simulink library "myLibrary"  (R2023b)
settings: Solver=VariableStepAuto  StartTime=0.0  StopTime=10.0  RelTol=1e-3
undefined symbols (not defined in the file): Cac_n1, ctrl1, Da, Discrete, dtha, ee_sli_rtmsupport, FA, gcbh, Ha, Ini, init_DCline, init_IPC, init_line, init_load, init_SG, init_shunt, init_TH, init_trafo, init_VSC, initMachineBlocks, Ka, Lf, Llkd_pu, Llkq1_pu, magnitude, NET, P, plots_step, q0, Rac_n1, Radd, Rkd_pu, Rkq1_pu, Rload_add, sim_config, sps_rtmsupport, spsSteamTurbineModel, T_DC_NET, T_global, T_IPC, T_load, T_NET, T_SG, T_shunt, T_STATCOM, T_TH, T_trafo, T_VSC, Ts, tstep, Udiff_a, V1
libraries: spsSeriesRLCBranchLib x105, eeGeneralControl x72, $bdroot x70, spsCurrentMeasurementLib x48, spsParallelRLCBranchLib x39, spsVoltageMeasurementLib x33, spsControlledVoltageSourceLib x27, spsFirstOrderFilterLib x16, dspsigops x6, spsThreePhaseVIMeasurementLib x5, spsPLL3phLib x4, spsThreePhaseBreakerLib x3
(part 3 of 12)

== system myLibrary/SG_step ==
  Add : Sum  Inputs=-+
  Add1 : Sum
  Add2 : Sum  Inputs=+-
  Bus Selector : BusSelector  OutputSignals="Mechanical.Electromagnetic torque  Te (pu),dq0 components.Stator current  iq (pu),dq0 components.Stator current  id (pu),dq0 components.Field current  ifd (pu),dq0 components.Damper winding current  ikd (pu),dq0 components.Damper winding current  ikq1 (pu),dq0 components.Damper winding current  ikq2 (pu),dq0 components.Stator voltage  vq (pu),dq0 components.Stator voltage  vd (pu),Mechanical.Rotor angle deviation  d_theta (rad),Mechanical.Rotor speed  wm (pu),Mechanical.Rotor mechanical angle  theta (deg),Load angle   delta  (deg)"
  Constant4 : Constant  Value=[2/3 1/3; -1/3 1/3 ; -1/3 -2/3]
  Constant_pi1 : Constant  Value=pi/2
  Constant_pi2 : Constant  Value=-pi/2
  Current Measurement3 : spsCurrentMeasurementLib/Current Measurement  PhasorSimulation=off  OutputType=Complex  PSBequivalent=0
  Demux4 : Demux  Outputs=3
  Display : Display
  Display1 : Display
  Exciter : Subsystem
  Gain : Gain  Gain=T_SG.wb
  Gain1 : Gain  Gain=pi/180
  Gain2 : Gain  Gain=1/T_SG.Lmd_pu
  Gain3 : Gain  Gain=pi/180
  Governor-Turbine : Subsystem
  Integrator : Integrator
  Mux4 : Mux  Inputs=2
  PLL (3ph) : spsPLL3phLib/PLL (3ph)  Fmin=45  Par_Init=[0, 50]  ParK=[180, 3200, 1]  TcD=1e-4  MaxRateChangeFreq=12  FilterCutOffFreq=25  Ts=0  AGC=on
  PLL (3ph)1 : spsPLL3phLib/PLL (3ph)  Fmin=45  Par_Init=[initSG.theta_in, 50]  ParK=[180, 3200, 1]  TcD=1e-4  MaxRateChangeFreq=12  FilterCutOffFreq=25  Ts=0  AGC=on
  Pm : Step  Time=tstep_P  Before=initSG.Pm  After=initSG.Pm*(1+sim_config.DR)  SampleTime=1e-4
  SM1 : spsSynchronousMachinepuFundamentalLib/Synchronous Machine pu Fundamental  PresetModel=No  MechanicalLoad=Mechanical power Pm  ShowDetailedParameters=on  RotorType=Round  Units=per unit fundamental parameters  MeasurementBus=off  NominalParameters=initMachineBlocks{SGnum,1}  Stator=initMachineBlocks{SGnum,2}  Field=initMachineBlocks{SGnum,3}  Dampers2=initMachineBlocks{SGnum,4}  Dampers1="[ Rkd_pu   Llkd_pu  Rkq1_pu  Llkq1_pu]"  Mechanical=initMachineBlocks{SGnum,5}  PolePairs=1  InitialConditions=initMachineBlocks{SGnum,6}  SetSaturation=off  Saturation=[0.6404,0.7127,0.8441,0.9214,0.9956,1.082,1.19,1.316,1.457;0.7,0.7698,0.8872,0.9466,0.9969,1.046,1.1,1.151,1.201]  LoadFlowParameters=[1 5.55 0 0 0]  TsPowergui=0  TsBlock=-1  IterativeModel=Trapezoidal non iterative  IterativeDiscreteModel=Trapezoidal non iterative  BusType=PV  Pref=5.55  Qref=0  Qmin=-Inf  Qmax=Inf  PLF=0  QLF=0
  Scope{,1..2,4,6,10} (6 alike) : Scope
  Scope3 : Scope  NumInputPorts=3
  Scope5 : Scope  NumInputPorts=2
  Scope7 : Scope  NumInputPorts=2
  Series RLC Branch1 : spsSeriesRLCBranchLib/Series RLC Branch  LConnTagsString=__new0  RConnTagsString=__new0  BranchType=RL  Resistance=T_SG.Rtr*T_SG.Zbpu_l2g  Inductance=T_SG.Ltr*T_SG.Zbpu_l2g  SetiL0=off  InitialCurrent=initSG.Itr  Capacitance=P.C  Setx0=on  InitialVoltage=P.C  Measurements=None
  Series RLC Branch2 : PMComponent  DialogController=POWERSYS.PowerSysDialog  LoadFcn=sps_rtmsupport('LoadFcn',gcbh);  StartFcn=sps_rtmsupport('StartFcn',gcbh);  StopFcn=sps_rtmsupport('StopFcn',gcbh);  PhysicalDomain=powersysdomain  LeftPortType=p1  RightPortType=p1  LConnTagsString=__new0  RConnTagsString=__new0  mask(Series RLC Branch){BranchType=RL, Resistance=T_SG.Rtr*T_SG.Zbpu_l2g, Inductance=T_SG.Ltr*T_SG.Zbpu_l2g, SetiL0=off, InitialCurrent=initSG.Itr, Capacitance=P.C, Setx0=on, InitialVoltage=P.C, Measurements=None}
      mask prompts: BranchType "Branch type:"; Resistance "Resistance (Ohms):"; Inductance "Inductance (H):"; SetiL0 "Set the initial inductor current"; InitialCurrent "Inductor initial current (A):"; Capacitance "Capacitance (F):"; Setx0 "Set the initial capacitor voltage"; InitialVoltage "Capacitor initial voltage (V):"
      mask help:
      | Implements a series branch of RLC elements.
      | Use the 'Branch type' parameter to add or remove elements from the branch.
      mask init:
      | [s1,s2,s3,s4,r1,r2,l1,l2,c1,c2,c3,c4] = powericon('Series RLC Branch',Resistance,Inductance,Capacitance,BranchType);
      | powericon('RLCCback',gcb)
      | power_initmask();
      settings: LibrarySourceBlock=spsSeriesRLCBranchLib/Series RLC Branch  CopyFcn=sps_rtmsupport('CopyFcn',gcbh);  DeleteFcn=sps_rtmsupport('DeleteFcn',gcbh);  UndoDeleteFcn=sps_rtmsupport('UndoDeleteFcn',gcbh);  ModelCloseFcn=sps_rtmsupport('ModelCloseFcn',gcbh);  PreSaveFcn=sps_rtmsupport('PreSaveFcn',gcbh);  PostSaveFcn=sps_rtmsupport('PostSaveFcn',gcbh);  NameChangeFcn=sps_rtmsupport('NameChangeFcn',gcbh);  PreCopyFcn=sps_rtmsupport('PreCopyFcn',gcbh);  OpenFcn=sps_rtmsupport('OpenFcn',gcbh, [1 4 7 9]);  CloseFcn=sps_rtmsupport('CloseFcn',gcbh);  PreDeleteFcn=sps_rtmsupport('PreDeleteFcn',gcbh);
      mask Help: helpview(psbhelp);
      mask TypeOptions BranchType: RLC | R | L | C | RL | RC | LC | Open circuit
      mask Callback BranchType: powericon('RLCCback',gcb)
      mask Callback Resistance: powericon('RLCCback',gcb)
      mask Callback Inductance: powericon('RLCCback',gcb)
      mask Callback SetiL0: powericon('RLCCback',gcb)
      mask Callback Capacitance: powericon('RLCCback',gcb)
      mask Callback Setx0: powericon('RLCCback',gcb)
      mask TypeOptions Measurements: None | Branch voltage | Branch current | Branch voltage and current
      mask Display:
      | plot(s1,s2,s3,s4,r1,r2*1.5,l1,l2*1.5,c1,c2*1.5,c3,c4*1.5)
      | color('red')
      | port_label('LConn',1,'+')
  Series RLC Branch3 : PMComponent  DialogController=POWERSYS.PowerSysDialog  LoadFcn=sps_rtmsupport('LoadFcn',gcbh);  StartFcn=sps_rtmsupport('StartFcn',gcbh);  StopFcn=sps_rtmsupport('StopFcn',gcbh);  PhysicalDomain=powersysdomain  LeftPortType=p1  RightPortType=p1  LConnTagsString=__new0  RConnTagsString=__new0  mask(Series RLC Branch){BranchType=RL, Resistance=T_SG.Rtr*T_SG.Zbpu_l2g, Inductance=T_SG.Ltr*T_SG.Zbpu_l2g, SetiL0=off, InitialCurrent=initSG.Itr, Capacitance=P.C, Setx0=on, InitialVoltage=P.C, Measurements=None}
      mask prompts: BranchType "Branch type:"; Resistance "Resistance (Ohms):"; Inductance "Inductance (H):"; SetiL0 "Set the initial inductor current"; InitialCurrent "Inductor initial current (A):"; Capacitance "Capacitance (F):"; Setx0 "Set the initial capacitor voltage"; InitialVoltage "Capacitor initial voltage (V):"
      mask help:
      | Implements a series branch of RLC elements.
      | Use the 'Branch type' parameter to add or remove elements from the branch.
      mask init:
      | [s1,s2,s3,s4,r1,r2,l1,l2,c1,c2,c3,c4] = powericon('Series RLC Branch',Resistance,Inductance,Capacitance,BranchType);
      | powericon('RLCCback',gcb)
      | power_initmask();
      settings: LibrarySourceBlock=spsSeriesRLCBranchLib/Series RLC Branch  CopyFcn=sps_rtmsupport('CopyFcn',gcbh);  DeleteFcn=sps_rtmsupport('DeleteFcn',gcbh);  UndoDeleteFcn=sps_rtmsupport('UndoDeleteFcn',gcbh);  ModelCloseFcn=sps_rtmsupport('ModelCloseFcn',gcbh);  PreSaveFcn=sps_rtmsupport('PreSaveFcn',gcbh);  PostSaveFcn=sps_rtmsupport('PostSaveFcn',gcbh);  NameChangeFcn=sps_rtmsupport('NameChangeFcn',gcbh);  PreCopyFcn=sps_rtmsupport('PreCopyFcn',gcbh);  OpenFcn=sps_rtmsupport('OpenFcn',gcbh, [1 4 7 9]);  CloseFcn=sps_rtmsupport('CloseFcn',gcbh);  PreDeleteFcn=sps_rtmsupport('PreDeleteFcn',gcbh);
      mask Help: helpview(psbhelp);
      mask TypeOptions BranchType: RLC | R | L | C | RL | RC | LC | Open circuit
      mask Callback BranchType: powericon('RLCCback',gcb)
      mask Callback Resistance: powericon('RLCCback',gcb)
      mask Callback Inductance: powericon('RLCCback',gcb)
      mask Callback SetiL0: powericon('RLCCback',gcb)
      mask Callback Capacitance: powericon('RLCCback',gcb)
      mask Callback Setx0: powericon('RLCCback',gcb)
      mask TypeOptions Measurements: None | Branch voltage | Branch current | Branch voltage and current
      mask Display:
      | plot(s1,s2,s3,s4,r1,r2*1.5,l1,l2*1.5,c1,c2*1.5,c3,c4*1.5)
      | color('red')
      | port_label('LConn',1,'+')
  Sum : Sum  Inputs=++++
  Te : Scope
  Three-Phase Series RLC Branch4 : spsThreePhaseSeriesRLCBranchLib/Three-Phase Series RLC Branch  LConnTagsString=A|B|C  RConnTagsString=A|B|C  BranchType=R  Resistance=T_SG.Rsnb*T_SG.Zbpu_l2g  Inductance=NET.L1_2/2  Capacitance=1/0.0528/(2*pi*50)  Measurements=None
  Three-Phase V-I Measurement : spsThreePhaseVIMeasurementLib/Three-Phase V-I Measurement  VoltageMeasurement=phase-to-phase  SetLabelV=off  LabelV=Vpcc  Vpu=off  VpuLL=off  CurrentMeasurement=no  SetLabelI=off  LabelI=Iabc  Ipu=off  Pbase=100e6  Vbase=500e3  OutputType=Complex  PhasorSimulation=off  PSBequivalent=0
  Three-Phase V-I Measurement1 : spsThreePhaseVIMeasurementLib/Three-Phase V-I Measurement  VoltageMeasurement=phase-to-phase  SetLabelV=off  LabelV=Vtr  Vpu=off  VpuLL=off  CurrentMeasurement=no  SetLabelI=off  LabelI=Iabc  Ipu=off  Pbase=100e6  Vbase=500e3  OutputType=Complex  PhasorSimulation=off  PSBequivalent=0
  Unwrap : dspsigops/Unwrap  tol=pi  InputProcessing=Columns as channels (frame based)  running=off
  Unwrap1 : dspsigops/Unwrap  tol=pi  InputProcessing=Columns as channels (frame based)  running=off
  Unwrap2 : dspsigops/Unwrap  tol=pi  InputProcessing=Columns as channels (frame based)  running=off
  "Vector magnitude " : Subsystem
  Vf : Constant  Value=initSG.Vf
  deg2rad : Gain  Gain=pi/180
  isqd : Scope  NumInputPorts=2
  mtx4 : Product  Multiplication=Matrix(*)
  qd3 : $bdroot/qd transform  SystemSampleTime=-1  VariantActivationTime=update diagram  AllowFlexibleInterface=on  Latency=0  AutoFrameSizeCalculation=off
  v_ref : Step  Time=tstep_V  Before=initSG.Vref  After=initSG.Vref*(1+sim_config.DR)  SampleTime=1e-4
  vqd : Scope  NumInputPorts=3
  A : PMIOPort  Side=Right
  B : PMIOPort  Port=2  Side=Right
  C : PMIOPort  Port=3  Side=Right
  tag scope: V_fn_pcc=global, theta_SG1=global, w_SG1=global
  wires:
  Three-Phase V-I Measurement1/1 -> [Vtr]
  Three-Phase V-I Measurement/1 -> [Vpcc]
  Bus Selector/10 -> [d_theta], Add1/1, Scope/1  "<Rotor angle deviation  d_theta (rad)>"
  Bus Selector/7 -> [ikq2]  "<Damper winding current  ikq2 (pu)>"
  [Vtr] -> PLL (3ph)/1
  Gain2/1 -> Scope1/1, [ifd]
  Bus Selector/5 -> [ikd]  "<Damper winding current  ikd (pu)>"
  Bus Selector/3 -> isqd/2, [isd]  "<Stator current  id (pu)>"
  Bus Selector/11 -> [we], Gain/1  "<Rotor speed  wm (pu)>"
  Bus Selector/6 -> [ikq1]  "<Damper winding current  ikq1 (pu)>"
  [Vpcc] -> PLL (3ph)1/1
  Bus Selector/4 -> Gain2/1  "<Field current  ifd (pu)>"
  Bus Selector/8 -> "Vector magnitude "/1(Vq), vqd/1, [vq]  "<Stator voltage  vq (pu)>"
  Bus Selector/1 -> Te/1, [Te]  "<Electromagnetic torque  Te (pu)>"
  Bus Selector/9 -> "Vector magnitude "/2(Vd), vqd/2, [vd]  "<Stator voltage  vd (pu)>"
  Gain/1 -> Scope6/1, [w_SG1], Integrator/1
  Current Measurement3/1 -> Scope2/1  "a"
  "Vector magnitude "/1(V) -> vqd/3  "V"
  Unwrap1/1 -> Add/1
  SM1/1 -> Bus Selector/1
  Bus Selector/13 -> [delta], Gain1/1, Gain3/1  "<Load angle   delta  (deg)>"
  Bus Selector/12 -> deg2rad/1, [theta]  "<Rotor mechanical angle  theta (deg)>"
  Bus Selector/2 -> isqd/1, [isq]  "<Stator current  iq (pu)>"
  Add/1 -> Scope4/1, Sum/4  "theta_in"
  Integrator/1 -> Sum/2
  PLL (3ph)1/2 -> Unwrap/1
  PLL (3ph)/2 -> Unwrap1/1
  Unwrap/1 -> Add/2
  Constant_pi1/1 -> Add1/2
  Add1/1 -> Scope5/1  "d_theta"
  Gain3/1 -> Scope5/2  "load_angle"
  Gain1/1 -> Sum/3
  Constant_pi2/1 -> Sum/1
  Governor-Turbine/1(Pm) -> SM1/1
  [we] -> Governor-Turbine/2(wm)  "wm"
  Pm/1 -> Governor-Turbine/1(Pref)
  [d_theta] -> Governor-Turbine/3(d_theta)
  deg2rad/1 -> Unwrap2/1
  Unwrap2/1 -> Add2/2, Scope3/3, [theta_SG1]  "THETA MATLAB"
  [we] -> Exciter/4(Vsi1)
  [vd] -> Exciter/3(Vd)
  [ifd] -> Exciter/6(Ifd_pu)
  [Te] -> Exciter/5(Vsi2)
  Vf/1 -> Exciter/7(Efd0_pu)
  v_ref/1 -> Exciter/1(V_REF)
  Exciter/1(Out1) -> SM1/2
  [vq] -> Exciter/2(Vq)
  Sum/1 -> Scope3/2, Add2/1  "OUR CALC"
  Add2/1 -> Scope3/1  "RESTA"
  qd3/1 -> Display/1, Scope7/1
  Demux4/1 -> Mux4/1
  [Vpcc] -> Demux4/1
  [V_fn_pcc] -> qd3/1
  Constant4/1 -> mtx4/1
  Demux4/2 -> Mux4/2
  Mux4/1 -> mtx4/2
  mtx4/1 -> [V_fn_pcc], Scope10/1
  qd3/2 -> Display1/1, Scope7/2
  [theta_SG1] -> qd3/2
  connections:
  Three-Phase V-I Measurement/LConn3 -- SM1/RConn3
  SM1/RConn2 -- Three-Phase V-I Measurement/LConn2
  Three-Phase V-I Measurement/LConn1 -- SM1/RConn1
  B/RConn1 -- Three-Phase V-I Measurement1/RConn2
  Series RLC Branch3/RConn1 -- Three-Phase V-I Measurement1/LConn3
  Series RLC Branch1/RConn1 -- Three-Phase V-I Measurement1/LConn1
  Current Measurement3/RConn1 -- Three-Phase Series RLC Branch4/RConn1
  A/RConn1 -- Three-Phase V-I Measurement1/RConn1
  C/RConn1 -- Three-Phase V-I Measurement1/RConn3
  Series RLC Branch2/RConn1 -- Three-Phase V-I Measurement1/LConn2
  Three-Phase V-I Measurement/RConn1 -- Series RLC Branch1/LConn1 -- Current Measurement3/LConn1
  Three-Phase V-I Measurement/RConn3 -- Series RLC Branch3/LConn1 -- Three-Phase Series RLC Branch4/RConn3
  Three-Phase Series RLC Branch4/LConn3 -- Three-Phase Series RLC Branch4/LConn2 -- Three-Phase Series RLC Branch4/LConn1
  Three-Phase V-I Measurement/RConn2 -- Series RLC Branch2/LConn1 -- Three-Phase Series RLC Branch4/RConn2

== system myLibrary/STATCOM ==
  Constant5 : Constant  Value=[ 2/3 1/3; -1/3 1/3 ; -1/3 -2/3]
  Control : Subsystem
      settings: PortSchema="{\"entries\":[{\"content\":{\"sides\":[{\"content\":{},\"type\":\"ConnectorPlacement.EquallySpacedRectSide\",\"uuid\":\"681c0b5f-022d-4b6d-8fe2-73940743a76e\"},{\"content\":{\"side\":\"RIGHT\"},\"type\":\"ConnectorPlacement.EquallySpacedRectSide\",\"uuid\":\"e9b400c8-e13f-4caf-91a1-f348979675fd\"},{\"content\":{\"connectorIds\":[\"In1\",\"Out1\",\"Out2\"],\"side\":\"TOP\"},\"type\":\"ConnectorPlacement.EquallySpacedRectSide\",\"uuid\":\"348007cb-ce67-4c45-ad7b-36ba89db6185\"},{\"content\":{\"connectorIds\":[\"In2\",\"In3\",\"In4\"],\"side\":\"BOTTOM\"},\"type\":\"ConnectorPlacement.EquallySpacedRectSide\",\"uuid\":\"fd6a847a-5d69-44cd-a0d1-495126761350\"}]},\"type\":\"ConnectorPlacement.EquallySpacedConnector\",\"uuid\":\"d16b8cae-5ced-4c76-a87e-983e154fb48f\"}],\"packageUris\":[\"http://schema.mathworks.com/mf0/Connector/R2020b\"],\"version\":\"1.0\"}"
  Current Measurement20 : spsCurrentMeasurementLib/Current Measurement  PhasorSimulation=off  OutputType=Complex  PSBequivalent=0
  Current Measurement21 : spsCurrentMeasurementLib/Current Measurement  PhasorSimulation=off  OutputType=Complex  PSBequivalent=0
  Current Measurement25 : spsCurrentMeasurementLib/Current Measurement  PhasorSimulation=off  OutputType=Complex  PSBequivalent=0
  Electrical : Subsystem
  Ig_l2g : Gain  Gain=1/T_VSC.Ibpu_l2g
  Is_l2g : Gain  Gain=1/T_VSC.Ibpu_l2g
  Mux10 : Mux  Inputs=2
  Mux4 : Mux  Inputs=3
  Product4 : Product  Multiplication=Matrix(*)
  Scope : Scope  NumInputPorts=3
  Series RLC Branch1 : spsSeriesRLCBranchLib/Series RLC Branch  LConnTagsString=__new0  RConnTagsString=__new0  BranchType=RL  Resistance=initVSC.Rtr  Inductance=initVSC.Ltr  SetiL0=off  InitialCurrent=initVSC.Iga  Capacitance=P.C  Setx0=on  InitialVoltage=P.C  Measurements=None
  Series RLC Branch10 : spsSeriesRLCBranchLib/Series RLC Branch  LConnTagsString=__new0  RConnTagsString=__new0  BranchType=R  Resistance=initVSC.Rac  Inductance=Lf  SetiL0=off  InitialCurrent=0  Capacitance=Cac_n1  Setx0=on  InitialVoltage=vcini_n1  Measurements=None
  Series RLC Branch2 : spsSeriesRLCBranchLib/Series RLC Branch  LConnTagsString=__new0  RConnTagsString=__new0  BranchType=RL  Resistance=initVSC.Rtr  Inductance=initVSC.Ltr  SetiL0=on  InitialCurrent=initVSC.Igb  Capacitance=P.C  Setx0=on  InitialVoltage=P.C  Measurements=None
  Series RLC Branch3 : spsSeriesRLCBranchLib/Series RLC Branch  LConnTagsString=__new0  RConnTagsString=__new0  BranchType=RL  Resistance=initVSC.Rtr  Inductance=initVSC.Ltr  SetiL0=on  InitialCurrent=initVSC.Igc  Capacitance=P.C  Setx0=on  InitialVoltage=P.C  Measurements=None
  Series RLC Branch4 : spsSeriesRLCBranchLib/Series RLC Branch  LConnTagsString=__new0  RConnTagsString=__new0  BranchType=C  Resistance=Rac_n1  Inductance=Lf  SetiL0=off  InitialCurrent=0  Capacitance=initVSC.Cac  Setx0=on  InitialVoltage=initVSC.Ucap_b  Measurements=None
  Series RLC Branch5 : spsSeriesRLCBranchLib/Series RLC Branch  LConnTagsString=__new0  RConnTagsString=__new0  BranchType=C  Resistance=Rac_n1  Inductance=Lf  SetiL0=off  InitialCurrent=0  Capacitance=initVSC.Cac  Setx0=on  InitialVoltage=initVSC.Ucap_a  Measurements=None
  Series RLC Branch6 : spsSeriesRLCBranchLib/Series RLC Branch  LConnTagsString=__new0  RConnTagsString=__new0  BranchType=R  Resistance=initVSC.Rac  Inductance=Lf  SetiL0=off  InitialCurrent=0  Capacitance=Cac_n1  Setx0=on  InitialVoltage=vcini_n1  Measurements=None
  Series RLC Branch8 : spsSeriesRLCBranchLib/Series RLC Branch  LConnTagsString=__new0  RConnTagsString=__new0  BranchType=R  Resistance=initVSC.Rac  Inductance=Lf  SetiL0=off  InitialCurrent=0  Capacitance=Cac_n1  Setx0=on  InitialVoltage=vcini_n1  Measurements=None
  Series RLC Branch9 : spsSeriesRLCBranchLib/Series RLC Branch  LConnTagsString=__new0  RConnTagsString=__new0  BranchType=C  Resistance=Rac_n1  Inductance=Lf  SetiL0=off  InitialCurrent=0  Capacitance=initVSC.Cac  Setx0=on  InitialVoltage=initVSC.Ucap_c  Measurements=None
  U_g2l : Gain  Gain=1/T_VSC.Vbpu_l2g
  Vdiff_l2g : Gain  Gain=T_VSC.Vbpu_l2g
  Voltage Measurement{,1..4} (5 alike) : spsVoltageMeasurementLib/Voltage Measurement  PhasorSimulation=off  OutputType=Complex  PSBequivalent=0
  VA : PMIOPort  Side=Right
  VB : PMIOPort  Port=2  Side=Right
  VC : PMIOPort  Port=3  Side=Right
  wires:
  Voltage Measurement1/1 -> Mux10/2
  Constant5/1 -> Product4/1
  Mux10/1 -> Product4/2
  Voltage Measurement/1 -> Mux10/1
  Product4/1 -> U_g2l/1
  Control/1(Vdiff_abc) -> Vdiff_l2g/1
  Electrical/2(Is) -> Is_l2g/1
  Vdiff_l2g/1 -> Electrical/2(vdiff)
  Is_l2g/1 -> Control/3(Iss)
  U_g2l/1 -> Control/2(U)
  Current Measurement20/1 -> Mux4/2
  Current Measurement21/1 -> Mux4/1
  Mux4/1 -> Ig_l2g/1
  Current Measurement25/1 -> Mux4/3
  Ig_l2g/1 -> Control/1(ig_abc)
  Voltage Measurement3/1 -> Scope/2
  Voltage Measurement2/1 -> Scope/1
  Voltage Measurement4/1 -> Scope/3
  Control/2(Pac) -> Electrical/1(Pac)
  Electrical/1(Vdc) -> Control/4(Vdc)
  connections:
  VB/RConn1 -- Current Measurement20/RConn1
  Series RLC Branch1/LConn1 -- Series RLC Branch5/LConn1 -- Voltage Measurement2/LConn1 -- Voltage Measurement/LConn1 -- Electrical/LConn1
  Voltage Measurement1/LConn2 -- Series RLC Branch9/LConn1 -- Voltage Measurement4/LConn1 -- Series RLC Branch3/LConn1 -- Electrical/LConn3
  VA/RConn1 -- Current Measurement21/RConn1
  Voltage Measurement1/LConn1 -- Series RLC Branch4/LConn1 -- Voltage Measurement3/LConn1 -- Series RLC Branch2/LConn1 -- Voltage Measurement/LConn2 -- Electrical/LConn2
  Current Measurement25/RConn1 -- VC/RConn1
  Series RLC Branch1/RConn1 -- Current Measurement21/LConn1
  Series RLC Branch2/RConn1 -- Current Measurement20/LConn1
  Series RLC Branch3/RConn1 -- Current Measurement25/LConn1
  Voltage Measurement2/LConn2 -- Series RLC Branch6/LConn1 -- Series RLC Branch5/RConn1
  Voltage Measurement3/LConn2 -- Series RLC Branch4/RConn1 -- Series RLC Branch8/LConn1
  Voltage Measurement4/LConn2 -- Series RLC Branch10/LConn1 -- Series RLC Branch9/RConn1
  Series RLC Branch10/RConn1 -- Series RLC Branch8/RConn1 -- Series RLC Branch6/RConn1

== system myLibrary/TH ==
  note: Grid Thevenin
  Series RLC Branch : spsSeriesRLCBranchLib/Series RLC Branch  LConnTagsString=__new0  RConnTagsString=__new0  BranchType=RL  Resistance=T.R  Inductance=T.L  SetiL0=off  InitialCurrent=ini.Itha  Capacitance=1e-6  Setx0=off  InitialVoltage=0  Measurements=None
  Series RLC Branch1 : spsSeriesRLCBranchLib/Series RLC Branch  LConnTagsString=__new0  RConnTagsString=__new0  BranchType=RL  Resistance=T.R  Inductance=T.L  SetiL0=on  InitialCurrent=ini.Ithb  Capacitance=1e-6  Setx0=off  InitialVoltage=0  Measurements=None
  Series RLC Branch2 : spsSeriesRLCBranchLib/Series RLC Branch  LConnTagsString=__new0  RConnTagsString=__new0  BranchType=RL  Resistance=T.R  Inductance=T.L  SetiL0=on  InitialCurrent=ini.Ithc  Capacitance=1e-6  Setx0=off  InitialVoltage=0  Measurements=None
  Three-Phase Source : spsThreePhaseSourceLib/Three-Phase Source  InternalConnection=Y  VoltagePhases=off  Voltage=ini.Vmag  PhaseAngle=ini.angle*180/pi  Voltage_phases=[25e3 25e3 25e3]/sqrt(3)  PhaseAngles_phases=[0 -120 +120]  Frequency="T_global{T_global.Area == T.Area,\"fb\"}"  NonIdealSource=off  SpecifyImpedance=off  Resistance=0.8929  Inductance=16.58e-3  ShortCircuitLevel=100e6  BaseVoltage=25e3  XRratio=7  BusType=swing  Pref=10e3  Qref=0  Prefabc=[10e3, 10e3, 10e3]  Qrefabc=[0, 0, 0]  Qmin=-inf  Qmax=inf
  A : PMIOPort  Side=Right
  B : PMIOPort  Port=2  Side=Right
  C : PMIOPort  Port=3  Side=Right
  connections:
  Series RLC Branch1/LConn1 -- Three-Phase Source/RConn2
  Series RLC Branch/LConn1 -- Three-Phase Source/RConn1
  A/RConn1 -- Series RLC Branch/RConn1
  B/RConn1 -- Series RLC Branch1/RConn1
  Series RLC Branch2/LConn1 -- Three-Phase Source/RConn3
  C/RConn1 -- Series RLC Branch2/RConn1

== system myLibrary/TH_step ==
  note: Grid Thevenin
  Constant1 : Constant  Value="2*pi*T_global{T_global.Area == T.Area,\"fb\"}"
  Constant2 : Constant  Value=2*pi/3
  Controlled Voltage Source : spsControlledVoltageSourceLib/Controlled Voltage Source  Initialize=on  Source_Type=AC  Amplitude=ini.Vmag/sqrt(3)*sqrt(2)  Phase=ini.angle*180/pi  Frequency=T_global.f_Hz  Measurements=None
  Controlled Voltage Source3 : spsControlledVoltageSourceLib/Controlled Voltage Source  Initialize=on  Source_Type=AC  Amplitude=ini.Vmag/sqrt(3)*sqrt(2)  Phase=ini.angle*180/pi-120  Frequency=T_global.f_Hz  Measurements=None
  Controlled Voltage Source4 : spsControlledVoltageSourceLib/Controlled Voltage Source  Initialize=on  Source_Type=AC  Amplitude=ini.Vmag/sqrt(3)*sqrt(2)  Phase=ini.angle*180/pi+120  Frequency=T_global.f_Hz  Measurements=None
  Current Measurement : spsCurrentMeasurementLib/Current Measurement  PhasorSimulation=off  OutputType=Complex  PSBequivalent=0
  Current Measurement1 : spsCurrentMeasurementLib/Current Measurement  PhasorSimulation=off  OutputType=Complex  PSBequivalent=0
  Current Measurement2 : spsCurrentMeasurementLib/Current Measurement  PhasorSimulation=off  OutputType=Complex  PSBequivalent=0
  Ground : spsGroundLib/Ground  LConnTagsString=a
  Integrator : Integrator  InitialCondition=ini.angle
  Product : Product
  Product1 : Product
  Product2 : Product
  Scope1 : Scope
  Scope2 : Scope
  Scope3 : Scope  NumInputPorts=3
  Series RLC Branch : spsSeriesRLCBranchLib/Series RLC Branch  LConnTagsString=__new0  RConnTagsString=__new0  BranchType=RL  Resistance=T.R  Inductance=T.L  SetiL0=on  InitialCurrent=ini.Itha  Capacitance=1e-6  Setx0=off  InitialVoltage=0  Measurements=None
  Series RLC Branch1 : spsSeriesRLCBranchLib/Series RLC Branch  LConnTagsString=__new0  RConnTagsString=__new0  BranchType=RL  Resistance=T.R  Inductance=T.L  SetiL0=on  InitialCurrent=ini.Ithb  Capacitance=1e-6  Setx0=off  InitialVoltage=0  Measurements=None
  Series RLC Branch2 : spsSeriesRLCBranchLib/Series RLC Branch  LConnTagsString=__new0  RConnTagsString=__new0  BranchType=RL  Resistance=T.R  Inductance=T.L  SetiL0=on  InitialCurrent=ini.Ithc  Capacitance=1e-6  Setx0=off  InitialVoltage=0  Measurements=None
  Sin : Trigonometry
  Sin1 : Trigonometry
  Sin2 : Trigonometry
  Step : Step  Time=tstep  Before=ini.Vmag/sqrt(3)*sqrt(2)  After=V1/sqrt(3)*sqrt(2)  SampleTime=1e-4
  Sum : Sum  Inputs=+-
  Sum1 : Sum
  Voltage Measurement : spsVoltageMeasurementLib/Voltage Measurement  PhasorSimulation=off  OutputType=Complex  PSBequivalent=0
  Voltage Measurement1 : spsVoltageMeasurementLib/Voltage Measurement  PhasorSimulation=off  OutputType=Complex  PSBequivalent=0
  A : PMIOPort  Side=Right
  B : PMIOPort  Port=2  Side=Right
  C : PMIOPort  Port=3  Side=Right
  wires:
  Current Measurement2/1 -> Scope3/3
  Current Measurement1/1 -> Scope3/2
  Current Measurement/1 -> Scope3/1
  Voltage Measurement1/1 -> Scope2/1
  Voltage Measurement/1 -> Scope1/1
  Sum1/1 -> Sin2/1
  Sin/1 -> Product/1
  Product1/1 -> Controlled Voltage Source3/1
  Product/1 -> Controlled Voltage Source/1
  Sum/1 -> Sin1/1
  Sin1/1 -> Product1/1
  Step/1 -> Product2/2, Product1/2, Product/2
  Sin2/1 -> Product2/1
  Product2/1 -> Controlled Voltage Source4/1
  Constant1/1 -> Integrator/1
  Constant2/1 -> Sum1/2, Sum/2
  Integrator/1 -> Sum/1, Sum1/1, Sin/1
  connections:
  Current Measurement2/RConn1 -- C/RConn1
  Voltage Measurement1/LConn2 -- Controlled Voltage Source3/RConn1 -- Series RLC Branch1/LConn1
  Voltage Measurement1/LConn1 -- Controlled Voltage Source/RConn1 -- Series RLC Branch/LConn1
  Current Measurement1/RConn1 -- B/RConn1 -- Voltage Measurement/LConn2
  Current Measurement/RConn1 -- A/RConn1 -- Voltage Measurement/LConn1
  Series RLC Branch/RConn1 -- Current Measurement/LConn1
  Series RLC Branch1/RConn1 -- Current Measurement1/LConn1
  Controlled Voltage Source4/RConn1 -- Series RLC Branch2/LConn1
  Series RLC Branch2/RConn1 -- Current Measurement2/LConn1
  Controlled Voltage Source/LConn1 -- Controlled Voltage Source4/LConn1 -- Ground/LConn1 -- Controlled Voltage Source3/LConn1

== system myLibrary/Trafo ==
  Series RLC Branch1 : spsSeriesRLCBranchLib/Series RLC Branch  LConnTagsString=__new0  RConnTagsString=__new0  BranchType=RL  Resistance=T.R  Inductance=T.L  SetiL0=on  InitialCurrent=ini.Ia  Capacitance=P.C  Setx0=on  InitialVoltage=P.C  Measurements=None
  Series RLC Branch2 : spsSeriesRLCBranchLib/Series RLC Branch  LConnTagsString=__new0  RConnTagsString=__new0  BranchType=RL  Resistance=T.R  Inductance=T.L  SetiL0=on  InitialCurrent=ini.Ib  Capacitance=P.C  Setx0=on  InitialVoltage=P.C  Measurements=None
  Series RLC Branch3 : spsSeriesRLCBranchLib/Series RLC Branch  LConnTagsString=__new0  RConnTagsString=__new0  BranchType=RL  Resistance=T.R  Inductance=T.L  SetiL0=on  InitialCurrent=ini.Ic  Capacitance=P.C  Setx0=on  InitialVoltage=P.C  Measurements=None
  A1 : PMIOPort  Side=Left
  B1 : PMIOPort  Port=2  Side=Left
  C1 : PMIOPort  Port=3  Side=Left
  A2 : PMIOPort  Port=4  Side=Right
  B2 : PMIOPort  Port=5  Side=Right
  C2 : PMIOPort  Port=6  Side=Right
  connections:
  Series RLC Branch1/RConn1 -- A2/RConn1
  Series RLC Branch2/RConn1 -- B2/RConn1
  Series RLC Branch3/RConn1 -- C2/RConn1
  Series RLC Branch2/LConn1 -- B1/RConn1
  Series RLC Branch1/LConn1 -- A1/RConn1
  Series RLC Branch3/LConn1 -- C1/RConn1

== system myLibrary/qd transform ==
  abc : Inport
  angle : Inport  Port=2
  Demux8 : Demux  Outputs=3
  qd0 Transformation : Subsystem
  q : Outport
  d : Outport  Port=2
  wires:
  qd0 Transformation/1(q) -> q/1  "q"
  Demux8/1 -> qd0 Transformation/1(a)
  qd0 Transformation/2(d) -> d/1  "d"
  Demux8/2 -> qd0 Transformation/2(b)
  abc/1 -> Demux8/1
  Demux8/3 -> qd0 Transformation/3(c)
  angle/1 -> qd0 Transformation/4(Angle)

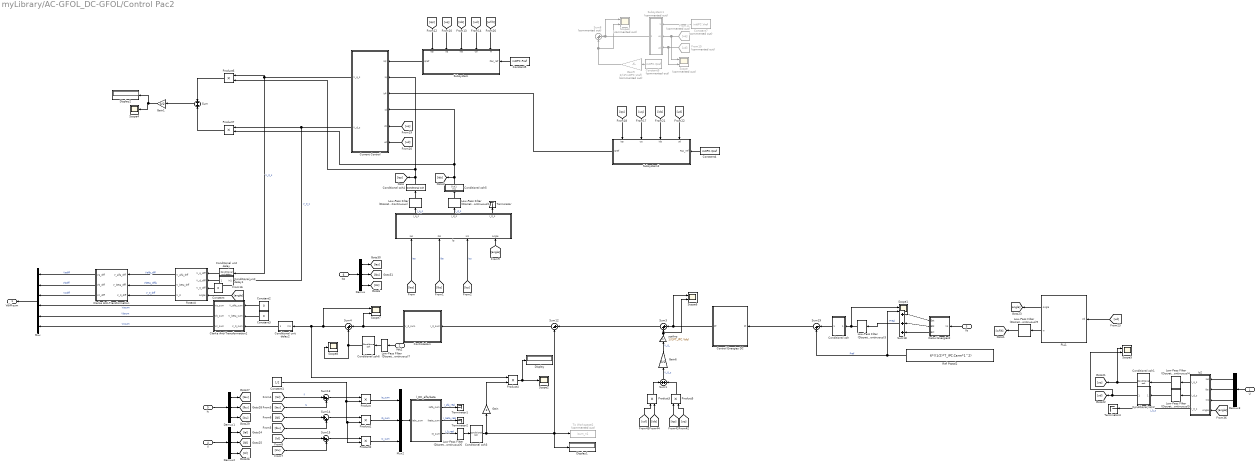
== system myLibrary/AC-GFOL_DC-GFOL/Control Pac2 ==
  U : Inport
  Vdc2 : Inport  Port=2
  Vs : Inport  Port=3
  Il : Inport  Port=4
  Iu : Inport  Port=5
  Iss : Inport  Port=6
  Calcul Energies2 : Subsystem
  Clarke Anti-Transformation : Subsystem
  Clarke Anti-Transformation2 : Subsystem
  Conditional unit delay : $bdroot/GFOL/Control/Conditional unit delay  SystemSampleTime=-1  VariantActivationTime=update diagram  AllowFlexibleInterface=on  Latency=0  AutoFrameSizeCalculation=off
      link override Constant4: Value=T_IPC.tau_cmd
      link override Unit Delay2: InitialCondition=initIPC.vdiffq  SampleTime=T_IPC.tau_cmd
  Conditional unit delay1 : Subsystem
  Conditional unit delay2 : Subsystem
  Conditional zoh : Subsystem
  Conditional zoh{1,3..4,6} (4 alike) : $bdroot/AC-GFOL_DC-GFOL/Control Pac2/Conditional zoh  SystemSampleTime=-1  VariantActivationTime=update diagram  AllowFlexibleInterface=on  Latency=0  AutoFrameSizeCalculation=off
  Conditional zoh2 : Subsystem
  Conditional zoh5 : Subsystem
  Constant : Constant  Value=0
  Constant1 : Constant  Value=1/2
  Constant2 : Constant  Value=0
  Constant3 : Constant  Value=0
  Constant4 : Constant  Value=initIPC.Qref
  Constant5 : Constant  Value=initIPC.Pref
  Constant7 : Constant  Commented=on  Value=initIPC.Vref
  Constant9 : Constant  Commented=on  Value=initIPC.Qref
  Control Energies DC : Subsystem
  Controladors : Subsystem
  Current Control : Subsystem
  Demux{,1..3} (4 alike) : Demux  Outputs=3
  Display : Display
  Display1 : Display
  Display2 : Display
  From11 : From  Commented=on  GotoTag=uq
  From15 : From  Commented=on  GotoTag=ud
  Gain : Gain  Gain=3
  Gain1 : Gain  Gain=3/2
  Gain6 : Gain  Gain=3/2
  Gain9 : Gain  Commented=on  Gain=2/(3*initIPC.Vref)
  Is : Subsystem
  Is2 : Subsystem
  Low-Pass Filter (Discrete or Continuous) : eeGeneralControl/Low-Pass Filter (Discrete or Continuous)  K=1  T=T_IPC.delay  B=inf  A=-inf  init_option=Specify as parameter  x0=initIPC.idiffq  Ts=0
  Low-Pass Filter (Discrete or Continuous)1 : eeGeneralControl/Low-Pass Filter (Discrete or Continuous)  K=1  T=T_IPC.delay  B=inf  A=-inf  init_option=Specify as parameter  x0=initIPC.idiffd  Ts=0
  Low-Pass Filter (Discrete or Continuous)3 : eeGeneralControl/Low-Pass Filter (Discrete or Continuous)  K=1  T=T_IPC.delay  B=inf  A=-inf  init_option=Specify as parameter  x0=6*((1/2)*T_IPC.Carm*1^2)  Ts=0
  Low-Pass Filter (Discrete or Continuous)4 : eeGeneralControl/Low-Pass Filter (Discrete or Continuous)  K=1  T=T_IPC.delay  B=inf  A=-inf  init_option=Specify as parameter  x0=initIPC.uq  Ts=0
  Low-Pass Filter (Discrete or Continuous)5 : eeGeneralControl/Low-Pass Filter (Discrete or Continuous)  K=1  T=T_IPC.delay  B=inf  A=-inf  init_option=Specify as parameter  x0=initIPC.ud  Ts=0
  Low-Pass Filter (Discrete or Continuous)6 : eeGeneralControl/Low-Pass Filter (Discrete or Continuous)  K=1  T=T_IPC.delay  B=inf  A=-inf  init_option=Specify as parameter  x0=initIPC.isum0_DC  Ts=0
  Low-Pass Filter (Discrete or Continuous)7 : eeGeneralControl/Low-Pass Filter (Discrete or Continuous)  K=1  T=T_IPC.delay  B=inf  A=-inf  init_option=Specify as parameter  x0=initIPC.Vdc  Ts=0
  Low-Pass Filter (Discrete or Continuous)9 : eeGeneralControl/Low-Pass Filter (Discrete or Continuous)  K=1  T=T_IPC.tw  B=inf  A=-inf  init_option=Specify as parameter  x0=2*pi*T_IPC.fb  Ts=0
  Mux : Mux  Inputs=6
  Mux2 : Mux  Inputs=3
  PLL1 : Subsystem
  Product{,1..7} (8 alike) : Product
  Ref Ptotal2 : Constant  Value=6*((1/2)*T_IPC.Carm*1^2)
  Rotació : Subsystem
  Scope : Scope  Commented=on  NumInputPorts=2
  Scope{1,5..7} (4 alike) : Scope  NumInputPorts=2
  Scope2 : Scope
  Scope3 : Scope  Commented=on  NumInputPorts=2
  Scope4 : Scope
  Scope8 : Scope
  Subsystem : Subsystem
      settings: PortSchema="{\"entries\":[{\"content\":{\"sides\":[{\"content\":{\"connectorIds\":[\"Out1\"]},\"type\":\"ConnectorPlacement.EquallySpacedRectSide\",\"uuid\":\"dea8424c-00e8-4bd8-a696-176e9d81b4b0\"},{\"content\":{\"connectorIds\":[\"In6\"],\"side\":\"RIGHT\"},\"type\":\"ConnectorPlacement.EquallySpacedRectSide\",\"uuid\":\"15b830a2-0897-480b-96a6-ff349e082a47\"},{\"content\":{\"connectorIds\":[\"In1\",\"In2\",\"In3\",\"In4\",\"In5\"],\"side\":\"TOP\"},\"type\":\"ConnectorPlacement.EquallySpacedRectSide\",\"uuid\":\"07916eec-e3fd-4ba3-9129-5b3a9aa06051\"}]},\"type\":\"ConnectorPlacement.EquallySpacedConnector\",\"uuid\":\"22000632-3c2a-414c-a4d7-471046f1c1a1\"}],\"packageUris\":[\"http://schema.mathworks.com/mf0/Connector/R2020b\"],\"version\":\"1.0\"}"
  Subsystem1 : Subsystem  Commented=on
      settings: PortSchema="{\"entries\":[{\"content\":{\"sides\":[{\"content\":{\"connectorIds\":[\"Out1\"]},\"type\":\"ConnectorPlacement.EquallySpacedRectSide\",\"uuid\":\"effe47ce-951a-4fb1-8fc1-e963775b8c82\"},{\"content\":{\"connectorIds\":[\"In1\",\"In2\",\"In3\"],\"side\":\"RIGHT\"},\"type\":\"ConnectorPlacement.EquallySpacedRectSide\",\"uuid\":\"a859b59d-6664-4e67-878a-4ecbefd8f8f0\"},{\"content\":{\"connectorIds\":[],\"side\":\"TOP\"},\"type\":\"ConnectorPlacement.EquallySpacedRectSide\",\"uuid\":\"0b762440-c8d9-40a7-a5db-13c46bc0406e\"}]},\"type\":\"ConnectorPlacement.EquallySpacedConnector\",\"uuid\":\"dbc4fef9-6b40-4568-97c6-19f27935f422\"}],\"packageUris\":[\"http://schema.mathworks.com/mf0/Connector/R2020b\"],\"version\":\"1.0\"}"
  Subsystem2 : Subsystem
      settings: PortSchema="{\"entries\":[{\"content\":{\"sides\":[{\"content\":{\"connectorIds\":[\"Out1\"]},\"type\":\"ConnectorPlacement.EquallySpacedRectSide\",\"uuid\":\"dea8424c-00e8-4bd8-a696-176e9d81b4b0\"},{\"content\":{\"connectorIds\":[\"In5\"],\"side\":\"RIGHT\"},\"type\":\"ConnectorPlacement.EquallySpacedRectSide\",\"uuid\":\"15b830a2-0897-480b-96a6-ff349e082a47\"},{\"content\":{\"connectorIds\":[\"In1\",\"In2\",\"In3\",\"In4\"],\"side\":\"TOP\"},\"type\":\"ConnectorPlacement.EquallySpacedRectSide\",\"uuid\":\"07916eec-e3fd-4ba3-9129-5b3a9aa06051\"}]},\"type\":\"ConnectorPlacement.EquallySpacedConnector\",\"uuid\":\"22000632-3c2a-414c-a4d7-471046f1c1a1\"}],\"packageUris\":[\"http://schema.mathworks.com/mf0/Connector/R2020b\"],\"version\":\"1.0\"}"
  Sum : Sum
  Sum1 : Sum
  Sum12 : Sum  Inputs=|+-
  Sum{3..4,13..15} (5 alike) : Sum  Inputs=|++
  Sum18 : Sum  Inputs=|+++
  Sum19 : Sum  Inputs=|-+
  Sum8 : Sum  Commented=on  Inputs=|++
  Terminator{,1..2,4} (4 alike) : Terminator
  To Workspace2 : ToWorkspace  Commented=on  VariableName=isum_n1  SampleTime=plots_step
  l_DC_alfa/beta : Subsystem
  scaling : Gain  Gain=1/(3*T_IPC.Vdc)
  Vdiff-sum : Outport
  wires:
  [wfilt] -> Subsystem/5(w)
  Low-Pass Filter (Discrete or Continuous)9/1 -> [wfilt]
  PLL1/2(w) -> Low-Pass Filter (Discrete or Continuous)9/1
  Low-Pass Filter (Discrete or Continuous)6/1 -> Conditional zoh3/1
  Is/3(I_0_s) -> Terminator/1
  Low-Pass Filter (Discrete or Continuous)7/1 -> Conditional zoh6/1
  Low-Pass Filter (Discrete or Continuous)5/1 -> Conditional zoh2/1(In1)
  Low-Pass Filter (Discrete or Continuous)1/1 -> Conditional zoh5/1(In1)
  Low-Pass Filter (Discrete or Continuous)/1 -> Conditional zoh4/1
  Ref Ptotal2/1 -> Sum19/2, Scope1/2  "Pref"
  Calcul Energies2/1(Eat) -> Sum18/1
  Constant2/1 -> Clarke Anti-Transformation2/1(V_alfa_sum)
  Constant3/1 -> Clarke Anti-Transformation2/2(V_beta_sum)
  Mux/1 -> Vdiff-sum/1
  Clarke Anti-Transformation2/1(Va_sum) -> Mux/4  "Vasum"
  Clarke Anti-Transformation2/2(Vb_sum) -> Mux/5  "Vbsum"
  Clarke Anti-Transformation/3(Vc_diff) -> Mux/3  "Vcdiff"
  Clarke Anti-Transformation/2(Vb_diff) -> Mux/2  "Vbdiff"
  Clarke Anti-Transformation/1(Va_diff) -> Mux/1  "Vadiff"
  Rotació/1(V_alfa_diff) -> Clarke Anti-Transformation/1(V_alfa_diff)  "Valfa_diff"
  Rotació/3(V_0) -> Clarke Anti-Transformation/3(V_0_diff)  "V_0_diff"
  [Ias] -> Is/1(Ias)  "Ias"
  [Ics] -> Is/3(Ics)  "Ics"
  [Ibs] -> Is/2(Ibs)  "Ibs"
  Rotació/2(V_beta_diff) -> Clarke Anti-Transformation/2(V_beta_dfff)  "Vbeta_diffa"
  Mux2/1 -> l_DC_alfa/beta/1(Iabc_sum)
  Product/1 -> Mux2/1  "Ia_sum"
  [Ial] -> Sum13/1  "Il"
  [Iau] -> Sum13/2  "Iu"
  Sum13/1 -> Product/1
  Constant1/1 -> Product2/2, Product1/2, Product/2
  Product1/1 -> Mux2/2  "Ib_sum"
  [Ibl] -> Sum14/1
  [Ibu] -> Sum14/2
  Sum14/1 -> Product1/1
  Product2/1 -> Mux2/3  "Ic_sum"
  [Icl] -> Sum15/1
  [Icu] -> Sum15/2
  Sum15/1 -> Product2/1
  Clarke Anti-Transformation2/3(Vc_sum) -> Mux/6  "Vcsum"
  Iu/1 -> Demux1/1
  Demux2/2 -> [Ibl]
  Demux1/1 -> [Iau]
  Demux1/3 -> [Icu]
  Il/1 -> Demux2/1
  Demux2/3 -> [Icl]
  Demux2/1 -> [Ial]
  Demux1/2 -> [Ibu]
  Demux3/2 -> Is2/2(Ibs)
  [angle] -> Is2/4(Angle)
  PLL1/1(Angle) -> [angle]
  [ud] -> PLL1/1(Ud)
  U/1 -> Demux3/1
  Demux3/3 -> Is2/3(Ics)
  Demux3/1 -> Is2/1(Ias)
  Demux/1 -> [Ias]
  Demux/2 -> [Ibs]
  Demux/3 -> [Ics]
  Iss/1 -> Demux/1
  Vs/1 -> Calcul Energies2/1(Vs)
  Calcul Energies2/3(Ect) -> Sum18/3
  Calcul Energies2/2(Ebt) -> Sum18/2
  [angle] -> Is/4(Angle)
  [angle] -> Rotació/4(Angle)
  Current Control/1(V_q_s) -> Product6/1, Conditional unit delay/1  "V_0_s"
  [uq] -> Current Control/5(uq)
  [ud] -> Current Control/6(ud)
  Controladors/1(V_0_sum) -> Scope7/2, Sum4/1
  Sum12/1 -> Controladors/1(I_0_sum)
  Sum19/1 -> Control Energies DC/1(Pt)
  [uq] -> Subsystem/2(uq)
  [iqs] -> Subsystem/1(iqs)
  [ud] -> Subsystem/4(ud)
  [ids] -> Subsystem/3(ids)
  Constant7/1 -> Subsystem1/1(uref)
  From11/1 -> Scope/1, Subsystem1/2(uq)
  From15/1 -> Scope/2, Subsystem1/3(ud)
  Is2/3(I_0_s) -> Terminator4/1  "I_0_s"
  Constant5/1 -> Subsystem/6(Pac_ref)
  Subsystem/1(iqref) -> Current Control/1(Iq*)
  [ud] -> Product3/1
  [uq] -> Product5/2
  Gain6/1 -> scaling/1  "V_0_"
  Sum1/1 -> Gain6/1  "V_0_s"
  Product5/1 -> Sum1/2
  Control Energies DC/1(Pt') -> Scope6/1, Sum3/1
  [iqs] -> Product5/1
  scaling/1 -> Scope6/2, Sum3/2
  Sum3/1 -> Sum12/1
  Product3/1 -> Sum1/1
  [ids] -> Product3/2
  Subsystem1/1(idref) -> Scope3/1, Sum8/1
  Constant9/1 -> Gain9/1
  Gain9/1 -> Scope3/2, Sum8/2
  Current Control/2(V_d_s) -> Product7/1, Conditional unit delay1/1(In1)  "V_0_s"
  Constant/1 -> Rotació/3(V_0_diff)
  l_DC_alfa/beta/1(Ialfa_sum) -> Terminator1/1  "I_afa_real"
  l_DC_alfa/beta/2(Ibeta_sum) -> Terminator2/1  "I_beta_real"
  Product4/1 -> Display/1, Scope2/1
  Gain/1 -> Product4/2
  Sum/1 -> Gain1/1
  Product6/1 -> Sum/1
  Product7/1 -> Sum/2
  Gain1/1 -> Display2/1, Scope4/1
  Constant4/1 -> Subsystem2/5(Pac_ref)
  [ids] -> Subsystem2/3(ids)
  [ud] -> Subsystem2/4(ud)
  [iqs] -> Subsystem2/1(iqs)
  [uq] -> Subsystem2/2(uq)
  Subsystem2/1(iqref) -> Current Control/3(Id*)
  Sum4/1 -> Scope7/1, Product4/1, Conditional unit delay2/1(In1)
  Conditional unit delay/1 -> Rotació/1(V_q_diff)
  Conditional unit delay1/1(Out1) -> Rotació/2(V_d_diff)
  Conditional unit delay2/1(Out1) -> Clarke Anti-Transformation2/3(V_0_sum)
  Is/1(I_q_s) -> Low-Pass Filter (Discrete or Continuous)/1  "I_q_s"
  Conditional zoh4/1 -> Product6/2, Current Control/2(Iq), [iqs]
  Is/2(I_d_s) -> Low-Pass Filter (Discrete or Continuous)1/1  "I_d_s"
  Conditional zoh5/1(Out1) -> Product7/2, Current Control/4(Id), [ids]
  Vdc2/1 -> Low-Pass Filter (Discrete or Continuous)7/1
  Conditional zoh6/1 -> Sum4/2, Scope8/1
  l_DC_alfa/beta/3(I0_sum) -> Low-Pass Filter (Discrete or Continuous)6/1  "I_0_real"
  Conditional zoh3/1 -> Gain/1, Display1/1, To Workspace2/1, Sum12/2
  Conditional zoh/1(Out1) -> Sum19/1
  Low-Pass Filter (Discrete or Continuous)3/1 -> Scope1/1, Conditional zoh/1(In1)
  Sum18/1 -> Low-Pass Filter (Discrete or Continuous)3/1  "Preal"
  Is2/1(I_q_s) -> Low-Pass Filter (Discrete or Continuous)4/1
  Low-Pass Filter (Discrete or Continuous)4/1 -> Conditional zoh1/1
  Conditional zoh1/1 -> Scope5/1, [uq]
  Conditional zoh2/1(Out1) -> Scope5/2, [ud]
  Is2/2(I_d_s) -> Low-Pass Filter (Discrete or Continuous)5/1

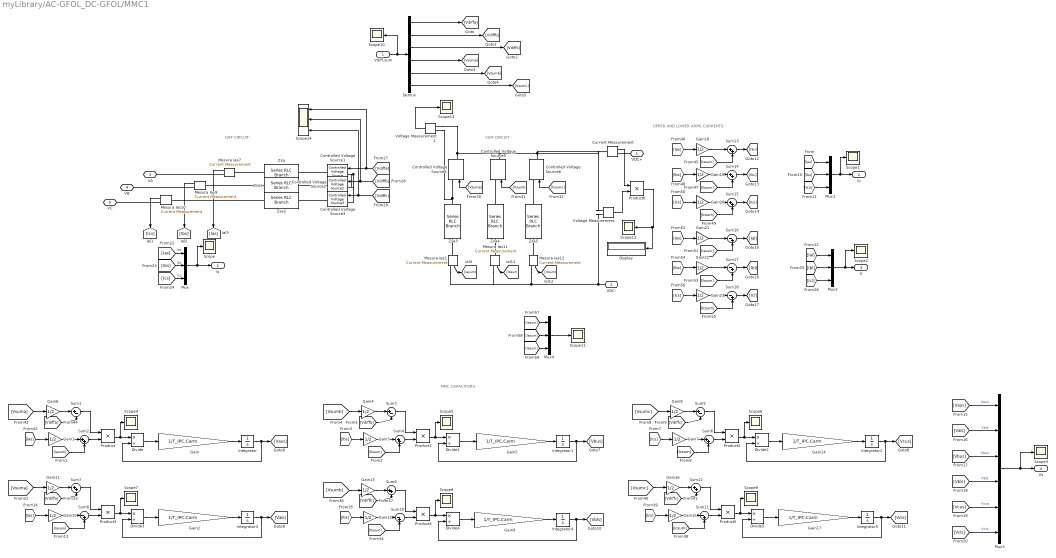
== system myLibrary/AC-GFOL_DC-GFOL/MMC1 ==
  note: UPPER AND LOWER ARMS CURRENTS:
  note: MMC CAPACITORS:
  note: SUM CIRCUIT:
  note: DIFF CIRCUIT:
  Vdiff,sum : Inport
  Controlled Voltage Source1 : spsControlledVoltageSourceLib/Controlled Voltage Source  Initialize=on  Source_Type=AC  Amplitude=initIPC.Udiff_mag  Phase=initIPC.angle_vdiff  Frequency=T_IPC.fb  Measurements=None
  Controlled Voltage Source2 : $bdroot/AC-GFOL_DC-GFOR/MMC1/Controlled Voltage Source2  Initialize=on  Source_Type=AC  Amplitude=initIPC.Udiff_mag  Phase=initIPC.angle_vdiff-120  Frequency=T_IPC.fb  Measurements=None
      settings: LibrarySourceBlock=spsControlledVoltageSourceLib/Controlled Voltage Source
  Controlled Voltage Source3 : $bdroot/AC-GFOL_DC-GFOR/MMC1/Controlled Voltage Source3  Initialize=on  Source_Type=AC  Amplitude=initIPC.Udiff_mag  Phase=initIPC.angle_vdiff+120  Frequency=T_IPC.fb  Measurements=None
      settings: LibrarySourceBlock=spsControlledVoltageSourceLib/Controlled Voltage Source
  Controlled Voltage Source4 : spsControlledVoltageSourceLib/Controlled Voltage Source  Initialize=on  Source_Type=DC  Amplitude=initIPC.Usuma  Phase=0  Frequency=0  Measurements=None
  Controlled Voltage Source5 : spsControlledVoltageSourceLib/Controlled Voltage Source  Initialize=on  Source_Type=DC  Amplitude=initIPC.Usumb  Phase=angle(Udiff_a)*180/pi  Frequency=60  Measurements=None
  Controlled Voltage Source6 : spsControlledVoltageSourceLib/Controlled Voltage Source  Initialize=on  Source_Type=DC  Amplitude=initIPC.Usumc  Phase=angle(Udiff_a)*180/pi  Frequency=60  Measurements=None
  Current Measurement : spsCurrentMeasurementLib/Current Measurement  PhasorSimulation=off  OutputType=Complex  PSBequivalent=0
  Demux : Demux  Outputs=6
  Display : Display
  Divide{,1..5} (6 alike) : Product  Inputs=*/
  Gain{,2,5,9,14,17} (6 alike) : Gain  Gain=1/T_IPC.Carm
  Gain{1,3..4,6..8,10..13,15..16,18..23} (18 alike) : Gain  Gain=1/2
  Integrator{,1..5} (6 alike) : Integrator  InitialCondition=1
  Mesura Ias{1,7,9..12} (6 alike) : spsCurrentMeasurementLib/Current Measurement  PhasorSimulation=off  OutputType=Complex  PSBequivalent=0
  Mux{,1..2,4} (4 alike) : Mux  Inputs=3
  Mux3 : Mux  Inputs=6
  Product{,1..6} (7 alike) : Product
  Scope{,1..13} (14 alike) : Scope
  Scope14 : Scope  NumInputPorts=3
  Sum1 : Sum  Inputs=|+-
  Sum{8,10..11,16..18} (6 alike) : Sum  Inputs=|-+
  Sum{2,4,6..7,9,12..15} (9 alike) : Sum  Inputs=|++
  Sum3 : Sum  Inputs=|+-
  Sum5 : Sum  Inputs=|+-
  Voltage Measurement : spsVoltageMeasurementLib/Voltage Measurement  PhasorSimulation=off  OutputType=Complex  PSBequivalent=0
  Voltage Measurement1 : spsVoltageMeasurementLib/Voltage Measurement  PhasorSimulation=off  OutputType=Complex  PSBequivalent=0
  Zsa : spsSeriesRLCBranchLib/Series RLC Branch  LConnTagsString=__new0  RConnTagsString=__new0  BranchType=RL  Resistance=T_IPC.Rc+T_IPC.Ra/2  Inductance=T_IPC.Lc+T_IPC.La/2  SetiL0=on  InitialCurrent=initIPC.Isa  Capacitance=1e-6  Setx0=off  InitialVoltage=0  Measurements=None
  Zsa1 : spsSeriesRLCBranchLib/Series RLC Branch  LConnTagsString=__new0  RConnTagsString=__new0  BranchType=RL  Resistance=T_IPC.Rc+T_IPC.Ra/2  Inductance=T_IPC.Lc+T_IPC.La/2  SetiL0=on  InitialCurrent=initIPC.Isb  Capacitance=1e-6  Setx0=off  InitialVoltage=0  Measurements=None
  Zsa2 : spsSeriesRLCBranchLib/Series RLC Branch  LConnTagsString=__new0  RConnTagsString=__new0  BranchType=RL  Resistance=T_IPC.Rc+T_IPC.Ra/2  Inductance=T_IPC.Lc+T_IPC.La/2  SetiL0=on  InitialCurrent=initIPC.Isc  Capacitance=1e-6  Setx0=off  InitialVoltage=0  Measurements=None
  Zsa3 : spsSeriesRLCBranchLib/Series RLC Branch  LConnTagsString=__new0  RConnTagsString=__new0  BranchType=RL  Resistance=2*T_IPC.Ra  Inductance=2*T_IPC.La  SetiL0=on  InitialCurrent=initIPC.isum0_DC  Capacitance=1e-6  Setx0=off  InitialVoltage=0  Measurements=None
  Zsa4 : spsSeriesRLCBranchLib/Series RLC Branch  LConnTagsString=__new0  RConnTagsString=__new0  BranchType=RL  Resistance=2*T_IPC.Ra  Inductance=2*T_IPC.La  SetiL0=on  InitialCurrent=initIPC.isum0_DC  Capacitance=1e-6  Setx0=off  InitialVoltage=0  Measurements=None
  Zsa5 : spsSeriesRLCBranchLib/Series RLC Branch  LConnTagsString=__new0  RConnTagsString=__new0  BranchType=RL  Resistance=2*T_IPC.Ra  Inductance=2*T_IPC.La  SetiL0=on  InitialCurrent=initIPC.isum0_DC  Capacitance=1e-6  Setx0=off  InitialVoltage=0  Measurements=None
  VDC+ : PMIOPort  Side=Right
  VDC- : PMIOPort  Port=2  Side=Right
  VA : PMIOPort  Port=3  Side=Left
  VB : PMIOPort  Port=4  Side=Left
  VC : PMIOPort  Port=5  Side=Left
  Is : Outport
  Iu : Outport  Port=2
  Il : Outport  Port=3
  Vs : Outport  Port=4
  wires:
  [Ibl] -> Mux2/2
  Sum18/1 -> [Icl]
  Gain23/1 -> Sum18/1
  [Ics] -> Gain23/1
  [Icsum] -> Sum18/2
  [Ibsum] -> Sum17/2
  [Ibs] -> Gain22/1
  Gain22/1 -> Sum17/1
  Sum17/1 -> [Ibl]
  Sum16/1 -> [Ial]
  Gain21/1 -> Sum16/1
  [Ias] -> Gain21/1
  [Iasum] -> Sum16/2
  Sum15/1 -> [Icu]
  [Icsum] -> Sum15/2
  Gain20/1 -> Sum15/1
  [Ics] -> Gain20/1
  [Ibs] -> Gain19/1
  Gain19/1 -> Sum14/1
  [Ibsum] -> Sum14/2
  Sum14/1 -> [Ibu]
  Sum13/1 -> [Iau]
  [Iasum] -> Sum13/2
  Gain18/1 -> Sum13/1
  [Ias] -> Gain18/1
  Sum11/1 -> Product5/2
  Product5/1 -> Scope9/1, Divide5/1
  Divide5/1 -> Gain17/1
  Gain17/1 -> Integrator5/1
  Integrator5/1 -> [Vcls], Divide5/2
  Gain16/1 -> Sum12/1
  [Vdiffc] -> Sum12/2
  [Icsum] -> Sum11/2
  Gain15/1 -> Sum11/1
  [Ics] -> Gain15/1
  [Vsumc] -> Gain16/1
  Sum12/1 -> Product5/1
  Sum9/1 -> Product4/1
  [Vsumb] -> Gain13/1
  [Ibs] -> Gain12/1
  Gain12/1 -> Sum10/1
  [Ibsum] -> Sum10/2
  [Vdiffb] -> Sum9/2
  Gain13/1 -> Sum9/1
  Integrator4/1 -> Divide4/2, [Vbls]
  Gain9/1 -> Integrator4/1
  Divide4/1 -> Gain9/1
  Product4/1 -> Divide4/1, Scope8/1
  Sum10/1 -> Product4/2
  Sum8/1 -> Product3/2
  Product3/1 -> Scope7/1, Divide3/1
  Divide3/1 -> Gain2/1
  Gain2/1 -> Integrator3/1
  Integrator3/1 -> [Vals], Divide3/2
  Gain11/1 -> Sum7/1
  [Vdiffa] -> Sum7/2
  [Iasum] -> Sum8/2
  Gain10/1 -> Sum8/1
  [Ias] -> Gain10/1
  [Vsuma] -> Gain11/1
  Sum7/1 -> Product3/1
  Sum5/1 -> Product2/1
  [Vsumc] -> Gain8/1
  [Ics] -> Gain7/1
  Gain7/1 -> Sum6/1
  [Icsum] -> Sum6/2
  [Vdiffc] -> Sum5/2
  Gain8/1 -> Sum5/1
  Integrator2/1 -> Divide2/2, [Vcus]
  Gain14/1 -> Integrator2/1
  Divide2/1 -> Gain14/1
  Product2/1 -> Divide2/1, Scope6/1
  Sum6/1 -> Product2/2
  Sum4/1 -> Product1/2
  Product1/1 -> Scope5/1, Divide1/1
  Divide1/1 -> Gain5/1
  Gain5/1 -> Integrator1/1
  Integrator1/1 -> [Vbus], Divide1/2
  Gain4/1 -> Sum3/1
  [Vdiffb] -> Sum3/2
  [Ibsum] -> Sum4/2
  Gain3/1 -> Sum4/1
  [Ibs] -> Gain3/1
  [Vsumb] -> Gain4/1
  Sum3/1 -> Product1/1
  Sum1/1 -> Product/1
  [Vsuma] -> Gain6/1
  [Ias] -> Gain1/1
  Gain1/1 -> Sum2/1
  [Iasum] -> Sum2/2
  [Vdiffa] -> Sum1/2
  Gain6/1 -> Sum1/1
  [Vsumc] -> Controlled Voltage Source6/1
  [Vsumb] -> Controlled Voltage Source5/1
  [Vsuma] -> Controlled Voltage Source4/1
  Mesura Ias12/1 -> [Icsum]
  Mesura Ias11/1 -> [Ibsum]
  Mesura Ias1/1 -> [Iasum]
  [Vdiffc] -> Scope14/3, Controlled Voltage Source3/1
  [Vdiffb] -> Scope14/2, Controlled Voltage Source2/1
  [Vdiffa] -> Scope14/1, Controlled Voltage Source1/1
  Integrator/1 -> Divide/2, [Vaus]
  Gain/1 -> Integrator/1
  Divide/1 -> Gain/1
  Product/1 -> Divide/1, Scope4/1
  Sum2/1 -> Product/2
  Mux3/1 -> Vs/1, Scope3/1
  [Vcls] -> Mux3/6  "Vcls"
  [Vcus] -> Mux3/5  "Vcus"
  [Vbls] -> Mux3/4  "Vbls"
  [Vbus] -> Mux3/3  "Vbus"
  [Vals] -> Mux3/2  "Vals"
  [Vaus] -> Mux3/1  "Vaus"
  [Icl] -> Mux2/3
  Mux2/1 -> Il/1, Scope2/1
  [Ial] -> Mux2/1
  Mux1/1 -> Iu/1, Scope1/1
  [Icu] -> Mux1/3
  [Ibu] -> Mux1/2
  [Iau] -> Mux1/1
  [Ias] -> Mux/1  "Ias"
  [Ibs] -> Mux/2  "Ibs"
  [Ics] -> Mux/3  "Ics"
  Mux/1 -> Is/1, Scope/1
  Demux/4 -> [Vsuma]
  Demux/2 -> [Vdiffb]
  Demux/3 -> [Vdiffc]
  Demux/1 -> [Vdiffa]
  Demux/6 -> [Vsumc]
  Demux/5 -> [Vsumb]
  Vdiff,sum/1 -> Scope10/1, Demux/1
  Mesura Ias9/1 -> [Ibs]
  Mesura Ias7/1 -> [Ias]
  Mesura Ias10/1 -> [Ics]
  [Iasum] -> Mux4/1
  [Iasum] -> Mux4/2
  [Iasum] -> Mux4/3
  Mux4/1 -> Scope11/1
  Current Measurement/1 -> Product6/1
  Voltage Measurement/1 -> Product6/2
  Product6/1 -> Display/1, Scope12/1
  Voltage Measurement1/1 -> Scope13/1
  connections:
  Mesura Ias12/RConn1 -- Mesura Ias11/RConn1 -- Mesura Ias1/RConn1 -- Voltage Measurement/LConn2 -- VDC-/RConn1
  Voltage Measurement/LConn1 -- Current Measurement/LConn1 -- Controlled Voltage Source6/RConn1 -- Controlled Voltage Source5/RConn1 -- Voltage Measurement1/LConn1 -- Controlled Voltage Source4/RConn1
  Controlled Voltage Source1/LConn1 -- Controlled Voltage Source3/LConn1 -- Controlled Voltage Source2/LConn1
  Controlled Voltage Source3/RConn1 -- Zsa2/LConn1
  Controlled Voltage Source2/RConn1 -- Zsa1/LConn1
  Controlled Voltage Source1/RConn1 -- Zsa/LConn1
  Zsa2/RConn1 -- Mesura Ias10/LConn1
  Zsa1/RConn1 -- Mesura Ias9/LConn1
  Zsa/RConn1 -- Mesura Ias7/LConn1
  Mesura Ias10/RConn1 -- VC/RConn1
  Mesura Ias9/RConn1 -- VB/RConn1
  Mesura Ias7/RConn1 -- VA/RConn1
  Zsa3/LConn1 -- Controlled Voltage Source4/LConn1 -- Voltage Measurement1/LConn2
  Zsa3/RConn1 -- Mesura Ias1/LConn1
  Zsa4/LConn1 -- Controlled Voltage Source5/LConn1
  Zsa4/RConn1 -- Mesura Ias11/LConn1
  Zsa5/LConn1 -- Controlled Voltage Source6/LConn1
  Zsa5/RConn1 -- Mesura Ias12/LConn1
  Current Measurement/RConn1 -- VDC+/RConn1
